simulink model "frbd_64ch_600mhz2"  (R2013b)
(part 3 of 138)

  bus_create0/1(bus_out) -> pipeline599/1(d)
  Constant123/1 -> adcsnap0/3(trig), adcsnap0/2(we)
  pipeline599/1(q) -> adcsnap0/1(din)
  Delay127/1 -> acc_cntrl10/2(sync)
  [acc_len] -> acc_cntrl10/1(acc_len)
  [cnt_rst] -> acc_cntrl10/3(rst)
  Constant124/1 -> acc_len/1(sim_1)
  acc_len/1(in_reg) -> pipeline600/1(d)
  pipeline600/1(q) -> [acc_len]
  Delay119/1 -> pipeline602/1(d)
  pipeline625/1(q) -> simple_bram_vacc86/1(new_acc)
  pipeline617/1(q) -> simple_bram_vacc86/2(din)
  pipeline624/1(q) -> Counter20/1
  acc_cntrl10/1(new_acc) -> pipeline605/1(d), pipeline607/1(d), pipeline603/1(d), pipeline625/1(d), pipeline624/1(d)
  pipeline602/1(q) -> pipeline617/1(d)
  simple_bram_vacc86/1(dout) -> Reinterpret80/1
  spec0/1(data_out) -> Terminator90/1
  Reinterpret80/1 -> spec0/2(data_in)
  simple_bram_vacc86/2(valid) -> Counter20/2, spec0/3(we)
  pipeline603/1(q) -> simple_bram_vacc40/1(new_acc)
  pipeline601/1(q) -> simple_bram_vacc40/2(din)
  simple_bram_vacc40/1(dout) -> Reinterpret81/1
  spec1/1(data_out) -> Terminator83/1
  Reinterpret81/1 -> spec1/2(data_in)
  simple_bram_vacc40/2(valid) -> spec1/3(we)
  pipeline607/1(q) -> simple_bram_vacc42/1(new_acc)
  pipeline606/1(q) -> simple_bram_vacc42/2(din)
  simple_bram_vacc42/1(dout) -> Reinterpret82/1
  spec2/1(data_out) -> Terminator85/1
  Reinterpret82/1 -> spec2/2(data_in)
  simple_bram_vacc42/2(valid) -> spec2/3(we)
  pipeline605/1(q) -> simple_bram_vacc41/1(new_acc)
  pipeline604/1(q) -> simple_bram_vacc41/2(din)
  simple_bram_vacc41/1(dout) -> Reinterpret83/1
  spec3/1(data_out) -> Terminator84/1
  Reinterpret83/1 -> spec3/2(data_in)
  simple_bram_vacc41/2(valid) -> spec3/3(we)
  Counter20/1 -> spec1/1(addr), spec3/1(addr), spec2/1(addr), spec0/1(addr)
  Delay120/1 -> pipeline616/1(d)
  pipeline616/1(q) -> pipeline601/1(d)
  Delay121/1 -> pipeline618/1(d)
  pipeline618/1(q) -> pipeline606/1(d)
  Delay122/1 -> pipeline619/1(d)
  pipeline619/1(q) -> pipeline604/1(d)
  asiaa_adc5g/16(c7) -> Terminator91/1
  asiaa_adc5g/15(c6) -> Terminator92/1
  asiaa_adc5g/14(c5) -> Terminator93/1
  asiaa_adc5g/13(c4) -> Terminator94/1
  asiaa_adc5g/12(c3) -> Terminator95/1
  asiaa_adc5g/11(c2) -> Terminator96/1
  asiaa_adc5g/10(c1) -> Terminator97/1
  asiaa_adc5g/9(c0) -> Terminator98/1
  Constant80/1 -> asiaa_adc5g/2(sim_c)
  Constant1/1 -> asiaa_adc5g/3(sim_sync)
  simple_bram_vacc1/2(valid) -> Terminator18/1
  simple_bram_vacc2/2(valid) -> Terminator1/1
  Constant81/1 -> asiaa_adc5g/1(sim_a)
  Delay5/1 -> acc_cntrl1/2(sync)
  [acc_len2] -> acc_cntrl1/1(acc_len)
  [cnt_rst] -> acc_cntrl1/3(rst)
  Delay8/1 -> pipeline52/1(d)
  pipeline39/1(q) -> simple_bram_vacc7/1(new_acc)
  pipeline30/1(q) -> simple_bram_vacc6/1(new_acc)
  pipeline27/1(q) -> simple_bram_vacc5/1(new_acc)
  pipeline44/1(q) -> simple_bram_vacc4/1(new_acc)
  pipeline12/1(q) -> simple_bram_vacc4/2(din)
  pipeline25/1(q) -> simple_bram_vacc5/2(din)
  pipeline28/1(q) -> simple_bram_vacc6/2(din)
  pipeline38/1(q) -> simple_bram_vacc7/2(din)
  pipeline40/1(q) -> Counter3/1
  simple_bram_vacc4/2(valid) -> pipeline45/1(d), Counter3/2
  simple_bram_vacc4/1(dout) -> Reinterpret4/1
  simple_bram_vacc5/1(dout) -> Reinterpret5/1
  simple_bram_vacc6/1(dout) -> Reinterpret6/1
  simple_bram_vacc7/1(dout) -> Reinterpret7/1
  Reinterpret4/1 -> pipeline43/1(d)
  Reinterpret5/1 -> pipeline46/1(d)
  Reinterpret6/1 -> pipeline47/1(d)
  Reinterpret7/1 -> pipeline48/1(d)
  Counter3/1 -> Relational5/2, Relational4/2
  Constant8/1 -> Mux6/2
  Constant15/1 -> Mux5/2
  Constant16/1 -> Mux7/2
  Constant17/1 -> Mux8/2
  AddSub3/1 -> AddSub5/1
  AddSub4/1 -> AddSub5/2
  pipeline54/1(q) -> pipeline55/1(d)
  edge_detect1/1 -> Logical3/1, Accumulator1/2
  pipeline53/1(q) -> Accumulator1/3, edge_detect1/1
  Slice2/1 -> Accumulator1/1
  Register1/1 -> frb_detector2/1(out_reg)
  [cnt_rst] -> Register1/2
  Relational3/1 -> Register1/1, Register1/3
  simple_bram_vacc7/2(valid) -> Terminator6/1
  pipeline45/1(q) -> Logical4/1, Mux5/1, Mux7/1, Mux8/1, pipeline56/1(d), Parallel_Dedispersor_v1/1(Valid)
  pipeline56/1(q) -> pipeline54/1(d)
  Accumulator1/1 -> Relational3/2, ACC2/2(data_in)
  Counter2/1 -> ACC2/1(addr)
  ACC2/1(data_out) -> Terminator7/1
  Logical3/1 -> Counter2/1
  Delay10/1 -> pipeline49/1(d)
  Delay14/1 -> pipeline50/1(d)
  Delay15/1 -> pipeline51/1(d)
  acc_cntrl1/1(new_acc) -> pipeline40/1(d), pipeline30/1(d), pipeline39/1(d), pipeline27/1(d), pipeline44/1(d)
  pipeline52/1(q) -> pipeline12/1(d)
  pipeline49/1(q) -> pipeline25/1(d)
  pipeline50/1(q) -> pipeline28/1(d)
  pipeline51/1(q) -> pipeline38/1(d)
  pipeline43/1(q) -> Mux6/3
  pipeline46/1(q) -> Mux5/3
  pipeline47/1(q) -> Mux7/3
  pipeline48/1(q) -> Mux8/3
  Mux6/1 -> Parallel_Dedispersor_v1/2(Data1)
  Mux5/1 -> Parallel_Dedispersor_v1/3(Data2)
  Mux7/1 -> Parallel_Dedispersor_v1/4(Data3)
  Mux8/1 -> Parallel_Dedispersor_v1/5(Data4)
  Parallel_Dedispersor_v1/1(Out1) -> pipeline57/1(d)
  Parallel_Dedispersor_v1/2(Out2) -> pipeline58/1(d)
  Parallel_Dedispersor_v1/3(Out3) -> pipeline59/1(d)
  Parallel_Dedispersor_v1/4(Out4) -> pipeline60/1(d)
  pipeline57/1(q) -> AddSub3/1
  pipeline58/1(q) -> AddSub3/2
  pipeline59/1(q) -> AddSub4/1
  pipeline60/1(q) -> AddSub4/2
  pipeline55/1(q) -> pipeline53/1(d)
  AddSub5/1 -> Slice2/1
  pipeline11/1(q) -> Logical4/3
  pipeline10/1(q) -> Logical4/2
  Logical4/1 -> Mux6/1
  Relational4/1 -> pipeline10/1(d)
  Relational5/1 -> pipeline11/1(d)
  Constant2/1 -> Relational4/1
  Constant9/1 -> Relational5/1
  Constant10/1 -> Logical3/2, ACC2/3(we)
  theta2/1(in_reg) -> Convert2/1
  Convert2/1 -> Relational3/1
  simple_bram_vacc5/2(valid) -> Terminator5/1
  simple_bram_vacc6/2(valid) -> Terminator4/1
  Delay19/1 -> acc_cntrl2/2(sync)
  [acc_len3] -> acc_cntrl2/1(acc_len)
  [cnt_rst] -> acc_cntrl2/3(rst)
  Delay21/1 -> pipeline92/1(d)
  pipeline73/1(q) -> simple_bram_vacc11/1(new_acc)
  pipeline71/1(q) -> simple_bram_vacc10/1(new_acc)
  pipeline69/1(q) -> simple_bram_vacc9/1(new_acc)
  pipeline76/1(q) -> simple_bram_vacc8/1(new_acc)
  pipeline66/1(q) -> simple_bram_vacc8/2(din)
  pipeline68/1(q) -> simple_bram_vacc9/2(din)
  pipeline70/1(q) -> simple_bram_vacc10/2(din)
  pipeline72/1(q) -> simple_bram_vacc11/2(din)
  pipeline74/1(q) -> Counter6/1
  simple_bram_vacc8/2(valid) -> pipeline77/1(d), Counter6/2
  simple_bram_vacc8/1(dout) -> Reinterpret8/1
  simple_bram_vacc9/1(dout) -> Reinterpret9/1
  simple_bram_vacc10/1(dout) -> Reinterpret10/1
  simple_bram_vacc11/1(dout) -> Reinterpret11/1
  Reinterpret8/1 -> pipeline75/1(d)
  Reinterpret9/1 -> pipeline78/1(d)
  Reinterpret10/1 -> pipeline80/1(d)
  Reinterpret11/1 -> pipeline83/1(d)
  Counter6/1 -> Relational8/2, Relational7/2
  Constant20/1 -> Mux10/2
  Constant33/1 -> Mux9/2
  Constant34/1 -> Mux11/2
  Constant35/1 -> Mux12/2
  AddSub6/1 -> AddSub8/1
  AddSub7/1 -> AddSub8/2
  pipeline97/1(q) -> pipeline98/1(d)
  edge_detect2/1 -> Logical5/1, Accumulator2/2
  pipeline93/1(q) -> Accumulator2/3, edge_detect2/1
  Slice3/1 -> Accumulator2/1
  Register2/1 -> frb_detector3/1(out_reg)
  [cnt_rst] -> Register2/2
  Relational6/1 -> Register2/1, Register2/3
  simple_bram_vacc11/2(valid) -> Terminator10/1
  pipeline77/1(q) -> Logical6/1, Mux9/1, Mux11/1, Mux12/1, pipeline119/1(d), Parallel_Dedispersor_v4/1(Valid)
  pipeline119/1(q) -> pipeline97/1(d)
  Accumulator2/1 -> Relational6/2, ACC3/2(data_in)
  Counter4/1 -> ACC3/1(addr)
  ACC3/1(data_out) -> Terminator11/1
  Logical5/1 -> Counter4/1
  Delay26/1 -> pipeline85/1(d)
  Delay27/1 -> pipeline90/1(d)
  Delay28/1 -> pipeline91/1(d)
  acc_cntrl2/1(new_acc) -> pipeline74/1(d), pipeline71/1(d), pipeline73/1(d), pipeline69/1(d), pipeline76/1(d)
  pipeline92/1(q) -> pipeline66/1(d)
  pipeline85/1(q) -> pipeline68/1(d)
  pipeline90/1(q) -> pipeline70/1(d)
  pipeline91/1(q) -> pipeline72/1(d)
  pipeline75/1(q) -> Mux10/3
  pipeline78/1(q) -> Mux9/3
  pipeline80/1(q) -> Mux11/3
  pipeline83/1(q) -> Mux12/3
  Mux10/1 -> Parallel_Dedispersor_v4/2(Data1)
  Mux9/1 -> Parallel_Dedispersor_v4/3(Data2)
  Mux11/1 -> Parallel_Dedispersor_v4/4(Data3)
  Mux12/1 -> Parallel_Dedispersor_v4/5(Data4)
  Parallel_Dedispersor_v4/1(Out1) -> pipeline120/1(d)
  Parallel_Dedispersor_v4/2(Out2) -> pipeline121/1(d)
  Parallel_Dedispersor_v4/3(Out3) -> pipeline122/1(d)
  Parallel_Dedispersor_v4/4(Out4) -> pipeline123/1(d)
  pipeline120/1(q) -> AddSub6/1
  pipeline121/1(q) -> AddSub6/2
  pipeline122/1(q) -> AddSub7/1
  pipeline123/1(q) -> AddSub7/2
  pipeline98/1(q) -> pipeline93/1(d)
  AddSub8/1 -> Slice3/1
  pipeline63/1(q) -> Logical6/3
  pipeline62/1(q) -> Logical6/2
  Logical6/1 -> Mux10/1
  Relational7/1 -> pipeline62/1(d)
  Relational8/1 -> pipeline63/1(d)
  Constant19/1 -> Relational7/1
  Constant21/1 -> Relational8/1
  Constant22/1 -> Logical5/2, ACC3/3(we)
  theta3/1(in_reg) -> Convert3/1
  Convert3/1 -> Relational6/1
  simple_bram_vacc9/2(valid) -> Terminator9/1
  simple_bram_vacc10/2(valid) -> Terminator8/1
  Delay29/1 -> acc_cntrl3/2(sync)
  [acc_len4] -> acc_cntrl3/1(acc_len)
  [cnt_rst] -> acc_cntrl3/3(rst)
  Delay30/1 -> pipeline110/1(d)
  pipeline95/1(q) -> simple_bram_vacc15/1(new_acc)
  pipeline84/1(q) -> simple_bram_vacc14/1(new_acc)
  pipeline81/1(q) -> simple_bram_vacc13/1(new_acc)
  pipeline100/1(q) -> simple_bram_vacc12/1(new_acc)
  pipeline65/1(q) -> simple_bram_vacc12/2(din)
  pipeline79/1(q) -> simple_bram_vacc13/2(din)
  pipeline82/1(q) -> simple_bram_vacc14/2(din)
  pipeline94/1(q) -> simple_bram_vacc15/2(din)
  pipeline96/1(q) -> Counter7/1
  simple_bram_vacc12/2(valid) -> Counter7/2, pipeline101/1(d)
  simple_bram_vacc12/1(dout) -> Reinterpret12/1
  simple_bram_vacc13/1(dout) -> Reinterpret13/1
  simple_bram_vacc14/1(dout) -> Reinterpret14/1
  simple_bram_vacc15/1(dout) -> Reinterpret15/1
  Reinterpret12/1 -> pipeline99/1(d)
  Reinterpret13/1 -> pipeline102/1(d)
  Reinterpret14/1 -> pipeline103/1(d)
  Reinterpret15/1 -> pipeline104/1(d)
  Counter7/1 -> Relational10/2, Relational11/2
  Constant36/1 -> Mux14/2
  Constant23/1 -> Mux13/2
  Constant24/1 -> Mux15/2
  Constant25/1 -> Mux16/2
  AddSub9/1 -> AddSub11/1
  AddSub10/1 -> AddSub11/2
  pipeline112/1(q) -> pipeline113/1(d)
  edge_detect3/1 -> Accumulator3/2, Logical7/1
  pipeline111/1(q) -> edge_detect3/1, Accumulator3/3
  Slice4/1 -> Accumulator3/1
  Register3/1 -> frb_detector4/1(out_reg)
  [cnt_rst] -> Register3/2
  Relational9/1 -> Register3/3, Register3/1
  simple_bram_vacc15/2(valid) -> Terminator14/1
  pipeline101/1(q) -> Parallel_Dedispersor_v3/1(Valid), pipeline114/1(d), Mux16/1, Mux15/1, Mux13/1, Logical8/1
  pipeline114/1(q) -> pipeline112/1(d)
  Accumulator3/1 -> ACC4/2(data_in), Relational9/2
  Counter5/1 -> ACC4/1(addr)
  ACC4/1(data_out) -> Terminator15/1
  Logical7/1 -> Counter5/1
  Delay18/1 -> pipeline105/1(d)
  Delay24/1 -> pipeline106/1(d)
  Delay25/1 -> pipeline107/1(d)
  acc_cntrl3/1(new_acc) -> pipeline100/1(d), pipeline81/1(d), pipeline95/1(d), pipeline84/1(d), pipeline96/1(d)
  pipeline110/1(q) -> pipeline65/1(d)
  pipeline105/1(q) -> pipeline79/1(d)
  pipeline106/1(q) -> pipeline82/1(d)
  pipeline107/1(q) -> pipeline94/1(d)
  pipeline99/1(q) -> Mux14/3
  pipeline102/1(q) -> Mux13/3
  pipeline103/1(q) -> Mux15/3
  pipeline104/1(q) -> Mux16/3
  Mux14/1 -> Parallel_Dedispersor_v3/2(Data1)
  Mux13/1 -> Parallel_Dedispersor_v3/3(Data2)
  Mux15/1 -> Parallel_Dedispersor_v3/4(Data3)
  Mux16/1 -> Parallel_Dedispersor_v3/5(Data4)
  Parallel_Dedispersor_v3/1(Out1) -> pipeline115/1(d)
  Parallel_Dedispersor_v3/2(Out2) -> pipeline116/1(d)
  Parallel_Dedispersor_v3/3(Out3) -> pipeline117/1(d)
  Parallel_Dedispersor_v3/4(Out4) -> pipeline118/1(d)
  pipeline115/1(q) -> AddSub9/1
  pipeline116/1(q) -> AddSub9/2
  pipeline117/1(q) -> AddSub10/1
  pipeline118/1(q) -> AddSub10/2
  pipeline113/1(q) -> pipeline111/1(d)
  AddSub11/1 -> Slice4/1
  pipeline64/1(q) -> Logical8/3
  pipeline61/1(q) -> Logical8/2
  Logical8/1 -> Mux14/1
  Relational10/1 -> pipeline61/1(d)
  Relational11/1 -> pipeline64/1(d)
  Constant32/1 -> Relational10/1
  Constant37/1 -> Relational11/1
  Constant18/1 -> ACC4/3(we), Logical7/2
  theta4/1(in_reg) -> Convert4/1
  Convert4/1 -> Relational9/1
  simple_bram_vacc13/2(valid) -> Terminator13/1
  simple_bram_vacc14/2(valid) -> Terminator12/1
  Delay32/1 -> acc_cntrl4/2(sync)
  [acc_len5] -> acc_cntrl4/1(acc_len)
  [cnt_rst] -> acc_cntrl4/3(rst)
  Delay39/1 -> pipeline178/1(d)
  pipeline163/1(q) -> simple_bram_vacc25/1(new_acc)
  pipeline161/1(q) -> simple_bram_vacc24/1(new_acc)
  pipeline159/1(q) -> simple_bram_vacc17/1(new_acc)
  pipeline166/1(q) -> simple_bram_vacc16/1(new_acc)
  pipeline157/1(q) -> simple_bram_vacc16/2(din)
  pipeline158/1(q) -> simple_bram_vacc17/2(din)
  pipeline160/1(q) -> simple_bram_vacc24/2(din)
  pipeline162/1(q) -> simple_bram_vacc25/2(din)
  pipeline164/1(q) -> Counter10/1
  simple_bram_vacc16/2(valid) -> pipeline167/1(d), Counter10/2
  simple_bram_vacc16/1(dout) -> Reinterpret16/1
  simple_bram_vacc17/1(dout) -> Reinterpret17/1
  simple_bram_vacc24/1(dout) -> Reinterpret24/1
  simple_bram_vacc25/1(dout) -> Reinterpret25/1
  Reinterpret16/1 -> pipeline165/1(d)
  Reinterpret17/1 -> pipeline168/1(d)
  Reinterpret24/1 -> pipeline170/1(d)
  Reinterpret25/1 -> pipeline173/1(d)
  Counter10/1 -> Relational16/2, Relational13/2
  Constant40/1 -> Mux25/2
  Constant61/1 -> Mux17/2
  Constant62/1 -> Mux26/2
  Constant63/1 -> Mux27/2
  AddSub12/1 -> AddSub16/1
  AddSub13/1 -> AddSub16/2
  pipeline183/1(q) -> pipeline184/1(d)
  edge_detect4/1 -> Logical9/1, Accumulator4/2
  pipeline179/1(q) -> Accumulator4/3, edge_detect4/1
  Slice5/1 -> Accumulator4/1
  Register4/1 -> frb_detector5/1(out_reg)
  [cnt_rst] -> Register4/2
  Relational12/1 -> Register4/1, Register4/3
  simple_bram_vacc25/2(valid) -> Terminator27/1
  pipeline167/1(q) -> Logical10/1, Mux17/1, Mux26/1, Mux27/1, pipeline209/1(d), Parallel_Dedispersor_v6/1(Valid)
  pipeline209/1(q) -> pipeline183/1(d)
  Accumulator4/1 -> Relational12/2, ACC5/2(data_in)
  Counter8/1 -> ACC5/1(addr)
  ACC5/1(data_out) -> Terminator28/1
  Logical9/1 -> Counter8/1
  Delay52/1 -> pipeline175/1(d)
  Delay53/1 -> pipeline176/1(d)
  Delay54/1 -> pipeline177/1(d)
  acc_cntrl4/1(new_acc) -> pipeline164/1(d), pipeline161/1(d), pipeline163/1(d), pipeline159/1(d), pipeline166/1(d)
  pipeline178/1(q) -> pipeline157/1(d)
  pipeline175/1(q) -> pipeline158/1(d)
  pipeline176/1(q) -> pipeline160/1(d)
  pipeline177/1(q) -> pipeline162/1(d)
  pipeline165/1(q) -> Mux25/3
  pipeline168/1(q) -> Mux17/3
  pipeline170/1(q) -> Mux26/3
  pipeline173/1(q) -> Mux27/3
  Mux25/1 -> Parallel_Dedispersor_v6/2(Data1)
  Mux17/1 -> Parallel_Dedispersor_v6/3(Data2)
  Mux26/1 -> Parallel_Dedispersor_v6/4(Data3)
  Mux27/1 -> Parallel_Dedispersor_v6/5(Data4)
  Parallel_Dedispersor_v6/1(Out1) -> pipeline228/1(d)
  Parallel_Dedispersor_v6/2(Out2) -> pipeline229/1(d)
  Parallel_Dedispersor_v6/3(Out3) -> pipeline230/1(d)
  Parallel_Dedispersor_v6/4(Out4) -> pipeline231/1(d)
  pipeline228/1(q) -> AddSub12/1
  pipeline229/1(q) -> AddSub12/2
  pipeline230/1(q) -> AddSub13/1
  pipeline231/1(q) -> AddSub13/2
  pipeline184/1(q) -> pipeline179/1(d)
  AddSub16/1 -> Slice5/1
  pipeline140/1(q) -> Logical10/3
  pipeline133/1(q) -> Logical10/2
  Logical10/1 -> Mux25/1
  Relational13/1 -> pipeline133/1(d)
  Relational16/1 -> pipeline140/1(d)
  Constant39/1 -> Relational13/1
  Constant41/1 -> Relational16/1
  Constant42/1 -> Logical9/2, ACC5/3(we)
  theta5/1(in_reg) -> Convert5/1
  Convert5/1 -> Relational12/1
  Delay3/1 -> Delay5/1, Delay19/1, Delay29/1, Delay32/1, Delay55/1, Delay43/1, Delay50/1, Delay58/1, Delay65/1, Delay127/1, Delay12/1
  simple_bram_vacc17/2(valid) -> Terminator26/1
  simple_bram_vacc24/2(valid) -> Terminator16/1
  power7/1 -> Delay15/1, Delay28/1, Delay25/1, Delay54/1, Delay41/1, Delay49/1, Delay46/1, Delay64/1, Delay61/1, Delay122/1, Delay37/1
  power5/1 -> Delay10/1, Delay26/1, Delay52/1, Delay31/1, Delay42/1, Delay62/1, Delay57/1, Delay120/1, Delay47/1, Delay18/1, Delay33/1
  Delay55/1 -> acc_cntrl5/2(sync)
  [acc_len6] -> acc_cntrl5/1(acc_len)
  [cnt_rst] -> acc_cntrl5/3(rst)
  Delay56/1 -> pipeline194/1(d)
  pipeline181/1(q) -> simple_bram_vacc29/1(new_acc)
  pipeline174/1(q) -> simple_bram_vacc28/1(new_acc)
  pipeline171/1(q) -> simple_bram_vacc27/1(new_acc)
  pipeline186/1(q) -> simple_bram_vacc26/1(new_acc)
  pipeline152/1(q) -> simple_bram_vacc26/2(din)
  pipeline169/1(q) -> simple_bram_vacc27/2(din)
  pipeline172/1(q) -> simple_bram_vacc28/2(din)
  pipeline180/1(q) -> simple_bram_vacc29/2(din)
  pipeline182/1(q) -> Counter11/1
  simple_bram_vacc26/2(valid) -> Counter11/2, pipeline187/1(d)
  simple_bram_vacc26/1(dout) -> Reinterpret26/1
  simple_bram_vacc27/1(dout) -> Reinterpret27/1
  simple_bram_vacc28/1(dout) -> Reinterpret28/1
  simple_bram_vacc29/1(dout) -> Reinterpret29/1
  Reinterpret26/1 -> pipeline185/1(d)
  Reinterpret27/1 -> pipeline188/1(d)
  Reinterpret28/1 -> pipeline189/1(d)
  Reinterpret29/1 -> pipeline190/1(d)
  Counter11/1 -> Relational18/2, Relational19/2
  Constant64/1 -> Mux29/2
  Constant43/1 -> Mux28/2
  Constant44/1 -> Mux30/2
  Constant45/1 -> Mux31/2
  AddSub17/1 -> AddSub19/1
  AddSub18/1 -> AddSub19/2
  pipeline196/1(q) -> pipeline197/1(d)
  edge_detect5/1 -> Accumulator5/2, Logical11/1
  pipeline195/1(q) -> edge_detect5/1, Accumulator5/3
  Slice6/1 -> Accumulator5/1
  Register5/1 -> frb_detector6/1(out_reg)
  [cnt_rst] -> Register5/2
  Relational17/1 -> Register5/3, Register5/1
  simple_bram_vacc29/2(valid) -> Terminator31/1
  pipeline187/1(q) -> Parallel_Dedispersor_v5/1(Valid), pipeline198/1(d), Mux31/1, Mux30/1, Mux28/1, Logical12/1
  pipeline198/1(q) -> pipeline196/1(d)
  Accumulator5/1 -> ACC6/2(data_in), Relational17/2
  Counter9/1 -> ACC6/1(addr)
  ACC6/1(data_out) -> Terminator32/1
  Logical11/1 -> Counter9/1
  Delay31/1 -> pipeline191/1(d)
  Delay40/1 -> pipeline192/1(d)
  Delay41/1 -> pipeline193/1(d)
  acc_cntrl5/1(new_acc) -> pipeline186/1(d), pipeline171/1(d), pipeline181/1(d), pipeline174/1(d), pipeline182/1(d)
  pipeline194/1(q) -> pipeline152/1(d)
  pipeline191/1(q) -> pipeline169/1(d)
  pipeline192/1(q) -> pipeline172/1(d)
  pipeline193/1(q) -> pipeline180/1(d)
  pipeline185/1(q) -> Mux29/3
  pipeline188/1(q) -> Mux28/3
  pipeline189/1(q) -> Mux30/3
  pipeline190/1(q) -> Mux31/3
  Mux29/1 -> Parallel_Dedispersor_v5/2(Data1)
  Mux28/1 -> Parallel_Dedispersor_v5/3(Data2)
  Mux30/1 -> Parallel_Dedispersor_v5/4(Data3)
  Mux31/1 -> Parallel_Dedispersor_v5/5(Data4)
  Parallel_Dedispersor_v5/1(Out1) -> pipeline199/1(d)
  Parallel_Dedispersor_v5/2(Out2) -> pipeline200/1(d)
  Parallel_Dedispersor_v5/3(Out3) -> pipeline201/1(d)
  Parallel_Dedispersor_v5/4(Out4) -> pipeline202/1(d)
  pipeline199/1(q) -> AddSub17/1
  pipeline200/1(q) -> AddSub17/2
  pipeline201/1(q) -> AddSub18/1
  pipeline202/1(q) -> AddSub18/2
  pipeline197/1(q) -> pipeline195/1(d)
  AddSub19/1 -> Slice6/1
  pipeline141/1(q) -> Logical12/3
  pipeline124/1(q) -> Logical12/2
  Logical12/1 -> Mux29/1
  Relational18/1 -> pipeline124/1(d)
  Relational19/1 -> pipeline141/1(d)
  Constant48/1 -> Relational18/1
  Constant65/1 -> Relational19/1
  Constant38/1 -> ACC6/3(we), Logical11/2
  theta6/1(in_reg) -> Convert6/1
  Convert6/1 -> Relational17/1
  simple_bram_vacc27/2(valid) -> Terminator30/1
  simple_bram_vacc28/2(valid) -> Terminator29/1
  Delay43/1 -> acc_cntrl6/2(sync)
  [acc_len7] -> acc_cntrl6/1(acc_len)
  [cnt_rst] -> acc_cntrl6/3(rst)
  Delay44/1 -> pipeline234/1(d)
  pipeline215/1(q) -> simple_bram_vacc19/1(new_acc)
  pipeline213/1(q) -> simple_bram_vacc18/1(new_acc)
  pipeline211/1(q) -> simple_bram_vacc31/1(new_acc)
  pipeline218/1(q) -> simple_bram_vacc30/1(new_acc)
  pipeline208/1(q) -> simple_bram_vacc30/2(din)
  pipeline210/1(q) -> simple_bram_vacc31/2(din)
  pipeline212/1(q) -> simple_bram_vacc18/2(din)
  pipeline214/1(q) -> simple_bram_vacc19/2(din)
  pipeline216/1(q) -> Counter14/1
  simple_bram_vacc30/2(valid) -> Counter14/2, pipeline219/1(d)
  simple_bram_vacc30/1(dout) -> Reinterpret30/1
  simple_bram_vacc31/1(dout) -> Reinterpret31/1
  simple_bram_vacc18/1(dout) -> Reinterpret18/1
  simple_bram_vacc19/1(dout) -> Reinterpret19/1
  Reinterpret30/1 -> pipeline217/1(d)
  Reinterpret31/1 -> pipeline220/1(d)
  Reinterpret18/1 -> pipeline222/1(d)
  Reinterpret19/1 -> pipeline225/1(d)
  Counter14/1 -> Relational21/2, Relational22/2
  Constant49/1 -> Mux18/2
  Constant56/1 -> Mux32/2
  Constant57/1 -> Mux19/2
  Constant58/1 -> Mux20/2
  AddSub20/1 -> AddSub22/1
  AddSub21/1 -> AddSub22/2
  pipeline239/1(q) -> pipeline240/1(d)
  edge_detect6/1 -> Accumulator6/2, Logical13/1
  pipeline235/1(q) -> edge_detect6/1, Accumulator6/3
  Slice7/1 -> Accumulator6/1
  Register6/1 -> frb_detector7/1(out_reg)
  [cnt_rst] -> Register6/2
  Relational20/1 -> Register6/3, Register6/1
  simple_bram_vacc19/2(valid) -> Terminator17/1
  pipeline219/1(q) -> Parallel_Dedispersor_v8/1(Valid), pipeline151/1(d), Mux20/1, Mux19/1, Mux32/1, Logical14/1
  pipeline151/1(q) -> pipeline239/1(d)
  Accumulator6/1 -> ACC7/2(data_in), Relational20/2
  Counter12/1 -> ACC7/1(addr)
  ACC7/1(data_out) -> Terminator19/1
  Logical13/1 -> Counter12/1
  Delay47/1 -> pipeline227/1(d)
  Delay48/1 -> pipeline232/1(d)
  Delay49/1 -> pipeline233/1(d)
  acc_cntrl6/1(new_acc) -> pipeline218/1(d), pipeline211/1(d), pipeline215/1(d), pipeline213/1(d), pipeline216/1(d)
  pipeline234/1(q) -> pipeline208/1(d)
  pipeline227/1(q) -> pipeline210/1(d)
  pipeline232/1(q) -> pipeline212/1(d)
  pipeline233/1(q) -> pipeline214/1(d)
  pipeline217/1(q) -> Mux18/3
  pipeline220/1(q) -> Mux32/3
  pipeline222/1(q) -> Mux19/3
  pipeline225/1(q) -> Mux20/3
  Mux18/1 -> Parallel_Dedispersor_v8/2(Data1)
  Mux32/1 -> Parallel_Dedispersor_v8/3(Data2)
  Mux19/1 -> Parallel_Dedispersor_v8/4(Data3)
  Mux20/1 -> Parallel_Dedispersor_v8/5(Data4)
  Parallel_Dedispersor_v8/1(Out1) -> pipeline153/1(d)
  Parallel_Dedispersor_v8/2(Out2) -> pipeline154/1(d)
  Parallel_Dedispersor_v8/3(Out3) -> pipeline155/1(d)
  Parallel_Dedispersor_v8/4(Out4) -> pipeline156/1(d)
  pipeline153/1(q) -> AddSub20/1
  pipeline154/1(q) -> AddSub20/2
  pipeline155/1(q) -> AddSub21/1
  pipeline156/1(q) -> AddSub21/2
  pipeline240/1(q) -> pipeline235/1(d)
  AddSub22/1 -> Slice7/1
  pipeline205/1(q) -> Logical14/3
  pipeline204/1(q) -> Logical14/2
  Logical14/1 -> Mux18/1
  Relational21/1 -> pipeline204/1(d)
  Relational22/1 -> pipeline205/1(d)
  Constant47/1 -> Relational21/1
  Constant50/1 -> Relational22/1
  Constant51/1 -> ACC7/3(we), Logical13/2
  theta7/1(in_reg) -> Convert7/1
  Convert7/1 -> Relational20/1
  simple_bram_vacc31/2(valid) -> Terminator34/1
  simple_bram_vacc18/2(valid) -> Terminator33/1
  Delay50/1 -> acc_cntrl7/2(sync)
  [acc_len8] -> acc_cntrl7/1(acc_len)
  [cnt_rst] -> acc_cntrl7/3(rst)
  Delay51/1 -> pipeline142/1(d)
  pipeline237/1(q) -> simple_bram_vacc23/1(new_acc)
  pipeline226/1(q) -> simple_bram_vacc22/1(new_acc)
  pipeline223/1(q) -> simple_bram_vacc21/1(new_acc)
  pipeline125/1(q) -> simple_bram_vacc20/1(new_acc)
  pipeline207/1(q) -> simple_bram_vacc20/2(din)
  pipeline221/1(q) -> simple_bram_vacc21/2(din)
  pipeline224/1(q) -> simple_bram_vacc22/2(din)
  pipeline236/1(q) -> simple_bram_vacc23/2(din)
  pipeline238/1(q) -> Counter15/1
  simple_bram_vacc20/2(valid) -> pipeline126/1(d), Counter15/2
  simple_bram_vacc20/1(dout) -> Reinterpret20/1
  simple_bram_vacc21/1(dout) -> Reinterpret21/1
  simple_bram_vacc22/1(dout) -> Reinterpret22/1
  simple_bram_vacc23/1(dout) -> Reinterpret23/1
  Reinterpret20/1 -> pipeline241/1(d)
  Reinterpret21/1 -> pipeline127/1(d)
  Reinterpret22/1 -> pipeline128/1(d)
  Reinterpret23/1 -> pipeline129/1(d)
  Counter15/1 -> Relational15/2, Relational14/2
  Constant59/1 -> Mux22/2
  Constant52/1 -> Mux21/2
  Constant53/1 -> Mux23/2
  Constant54/1 -> Mux24/2
  AddSub23/1 -> AddSub15/1
  AddSub14/1 -> AddSub15/2
  pipeline144/1(q) -> pipeline145/1(d)
  edge_detect7/1 -> Logical15/1, Accumulator7/2
  pipeline143/1(q) -> Accumulator7/3, edge_detect7/1
  Slice8/1 -> Accumulator7/1
  Register7/1 -> frb_detector8/1(out_reg)
  [cnt_rst] -> Register7/2
  Relational23/1 -> Register7/1, Register7/3
  simple_bram_vacc23/2(valid) -> Terminator24/1
  pipeline126/1(q) -> Logical16/1, Mux21/1, Mux23/1, Mux24/1, pipeline146/1(d), Parallel_Dedispersor_v7/1(Valid)
  pipeline146/1(q) -> pipeline144/1(d)
  Accumulator7/1 -> Relational23/2, ACC8/2(data_in)
  Counter13/1 -> ACC8/1(addr)
  ACC8/1(data_out) -> Terminator25/1
  Logical15/1 -> Counter13/1
  Delay42/1 -> pipeline130/1(d)
  Delay45/1 -> pipeline131/1(d)
  Delay46/1 -> pipeline132/1(d)
  acc_cntrl7/1(new_acc) -> pipeline238/1(d), pipeline226/1(d), pipeline237/1(d), pipeline223/1(d), pipeline125/1(d)
  pipeline142/1(q) -> pipeline207/1(d)
  pipeline130/1(q) -> pipeline221/1(d)
  pipeline131/1(q) -> pipeline224/1(d)
  pipeline132/1(q) -> pipeline236/1(d)
  pipeline241/1(q) -> Mux22/3
  pipeline127/1(q) -> Mux21/3
  pipeline128/1(q) -> Mux23/3
  pipeline129/1(q) -> Mux24/3
  Mux22/1 -> Parallel_Dedispersor_v7/2(Data1)
  Mux21/1 -> Parallel_Dedispersor_v7/3(Data2)
  Mux23/1 -> Parallel_Dedispersor_v7/4(Data3)
  Mux24/1 -> Parallel_Dedispersor_v7/5(Data4)
  Parallel_Dedispersor_v7/1(Out1) -> pipeline147/1(d)
  Parallel_Dedispersor_v7/2(Out2) -> pipeline148/1(d)
  Parallel_Dedispersor_v7/3(Out3) -> pipeline149/1(d)
  Parallel_Dedispersor_v7/4(Out4) -> pipeline150/1(d)
  pipeline147/1(q) -> AddSub23/1
  pipeline148/1(q) -> AddSub23/2
  pipeline149/1(q) -> AddSub14/1
  pipeline150/1(q) -> AddSub14/2
  pipeline145/1(q) -> pipeline143/1(d)
  AddSub15/1 -> Slice8/1
  pipeline206/1(q) -> Logical16/3
  pipeline203/1(q) -> Logical16/2
  Logical16/1 -> Mux22/1
  Relational14/1 -> pipeline203/1(d)
  Relational15/1 -> pipeline206/1(d)
  Constant55/1 -> Relational14/1
  Constant60/1 -> Relational15/1
  Constant46/1 -> Logical15/2, ACC8/3(we)
  theta8/1(in_reg) -> Convert8/1
  Convert8/1 -> Relational23/1
  simple_bram_vacc21/2(valid) -> Terminator23/1
  simple_bram_vacc22/2(valid) -> Terminator20/1
  Delay58/1 -> acc_cntrl8/2(sync)
  [acc_len9] -> acc_cntrl8/1(acc_len)
  [cnt_rst] -> acc_cntrl8/3(rst)
  Delay59/1 -> pipeline290/1(d)
  pipeline275/1(q) -> simple_bram_vacc33/1(new_acc)
  pipeline273/1(q) -> simple_bram_vacc32/1(new_acc)
  pipeline271/1(q) -> simple_bram_vacc39/1(new_acc)
  pipeline278/1(q) -> simple_bram_vacc38/1(new_acc)
  pipeline269/1(q) -> simple_bram_vacc38/2(din)
  pipeline270/1(q) -> simple_bram_vacc39/2(din)
  pipeline272/1(q) -> simple_bram_vacc32/2(din)
  pipeline274/1(q) -> simple_bram_vacc33/2(din)
  pipeline276/1(q) -> Counter18/1
  simple_bram_vacc38/2(valid) -> pipeline279/1(d), Counter18/2
  simple_bram_vacc38/1(dout) -> Reinterpret38/1
  simple_bram_vacc39/1(dout) -> Reinterpret39/1
  simple_bram_vacc32/1(dout) -> Reinterpret32/1
  simple_bram_vacc33/1(dout) -> Reinterpret33/1
  Reinterpret38/1 -> pipeline277/1(d)
  Reinterpret39/1 -> pipeline280/1(d)
  Reinterpret32/1 -> pipeline282/1(d)
  Reinterpret33/1 -> pipeline285/1(d)
  Counter18/1 -> Relational28/2, Relational27/2
  Constant68/1 -> Mux33/2
  Constant75/1 -> Mux40/2
  Constant76/1 -> Mux34/2
  Constant77/1 -> Mux35/2
  AddSub26/1 -> AddSub28/1
  AddSub27/1 -> AddSub28/2
  pipeline295/1(q) -> pipeline296/1(d)
  edge_detect8/1 -> Logical17/1, Accumulator8/2
  pipeline291/1(q) -> Accumulator8/3, edge_detect8/1
  Slice9/1 -> Accumulator8/1
  Register8/1 -> frb_detector9/1(out_reg)
  [cnt_rst] -> Register8/2
  Relational26/1 -> Register8/1, Register8/3
  simple_bram_vacc33/2(valid) -> Terminator35/1
  pipeline279/1(q) -> Mux40/1, Mux34/1, Mux35/1, pipeline259/1(d), Parallel_Dedispersor_v10/1(Valid), Logical18/1
  pipeline259/1(q) -> pipeline295/1(d)
  Accumulator8/1 -> Relational26/2, ACC9/2(data_in)
  Counter16/1 -> ACC9/1(addr)
  ACC9/1(data_out) -> Terminator36/1
  Logical17/1 -> Counter16/1
  Delay62/1 -> pipeline287/1(d)
  Delay63/1 -> pipeline288/1(d)
  Delay64/1 -> pipeline289/1(d)
  acc_cntrl8/1(new_acc) -> pipeline276/1(d), pipeline273/1(d), pipeline275/1(d), pipeline271/1(d), pipeline278/1(d)
  pipeline290/1(q) -> pipeline269/1(d)
  pipeline287/1(q) -> pipeline270/1(d)
  pipeline288/1(q) -> pipeline272/1(d)
  pipeline289/1(q) -> pipeline274/1(d)
  pipeline277/1(q) -> Mux33/3
  pipeline280/1(q) -> Mux40/3
  pipeline282/1(q) -> Mux34/3
  pipeline285/1(q) -> Mux35/3
  Mux33/1 -> Parallel_Dedispersor_v10/2(Data1)
  Mux40/1 -> Parallel_Dedispersor_v10/3(Data2)
  Mux34/1 -> Parallel_Dedispersor_v10/4(Data3)
  Mux35/1 -> Parallel_Dedispersor_v10/5(Data4)
  Parallel_Dedispersor_v10/1(Out1) -> pipeline260/1(d)
  Parallel_Dedispersor_v10/2(Out2) -> pipeline261/1(d)
  Parallel_Dedispersor_v10/3(Out3) -> pipeline262/1(d)
  Parallel_Dedispersor_v10/4(Out4) -> pipeline263/1(d)
  pipeline260/1(q) -> AddSub26/1
  pipeline261/1(q) -> AddSub26/2
  pipeline262/1(q) -> AddSub27/1
  pipeline263/1(q) -> AddSub27/2
  pipeline296/1(q) -> pipeline291/1(d)
  AddSub28/1 -> Slice9/1
  pipeline266/1(q) -> Logical18/3
  pipeline265/1(q) -> Logical18/2
  Logical18/1 -> Mux33/1
  Relational27/1 -> pipeline265/1(d)
  Relational28/1 -> pipeline266/1(d)
  Constant67/1 -> Relational27/1
  Constant69/1 -> Relational28/1
  Constant70/1 -> Logical17/2, ACC9/3(we)
  theta9/1(in_reg) -> Convert9/1
  Convert9/1 -> Relational26/1
  simple_bram_vacc39/2(valid) -> Terminator42/1
  simple_bram_vacc32/2(valid) -> Terminator41/1
  Delay65/1 -> acc_cntrl9/2(sync)
  [acc_len10] -> acc_cntrl9/1(acc_len)
  [cnt_rst] -> acc_cntrl9/3(rst)
  Delay66/1 -> pipeline250/1(d)
  pipeline293/1(q) -> simple_bram_vacc37/1(new_acc)
  pipeline286/1(q) -> simple_bram_vacc36/1(new_acc)
  pipeline283/1(q) -> simple_bram_vacc35/1(new_acc)
  pipeline242/1(q) -> simple_bram_vacc34/1(new_acc)
  pipeline268/1(q) -> simple_bram_vacc34/2(din)
  pipeline281/1(q) -> simple_bram_vacc35/2(din)
  pipeline284/1(q) -> simple_bram_vacc36/2(din)
  pipeline292/1(q) -> simple_bram_vacc37/2(din)
  pipeline294/1(q) -> Counter19/1
  simple_bram_vacc34/2(valid) -> Counter19/2, pipeline243/1(d)
  simple_bram_vacc34/1(dout) -> Reinterpret34/1
  simple_bram_vacc35/1(dout) -> Reinterpret35/1
  simple_bram_vacc36/1(dout) -> Reinterpret36/1
  simple_bram_vacc37/1(dout) -> Reinterpret37/1
  Reinterpret34/1 -> pipeline297/1(d)
  Reinterpret35/1 -> pipeline244/1(d)
  Reinterpret36/1 -> pipeline245/1(d)
  Reinterpret37/1 -> pipeline246/1(d)
  Counter19/1 -> Relational24/2, Relational25/2
  Constant78/1 -> Mux37/2
  Constant71/1 -> Mux36/2
  Constant72/1 -> Mux38/2
  Constant73/1 -> Mux39/2
  AddSub29/1 -> AddSub25/1
  AddSub24/1 -> AddSub25/2
  pipeline252/1(q) -> pipeline253/1(d)
  edge_detect9/1 -> Accumulator9/2, Logical19/1
  pipeline251/1(q) -> edge_detect9/1, Accumulator9/3
  Slice10/1 -> Accumulator9/1
  Register9/1 -> frb_detector10/1(out_reg)
  [cnt_rst] -> Register9/2
  Relational29/1 -> Register9/3, Register9/1
  simple_bram_vacc37/2(valid) -> Terminator39/1
  pipeline243/1(q) -> Parallel_Dedispersor_v9/1(Valid), pipeline254/1(d), Mux39/1, Mux38/1, Mux36/1, Logical20/1
  pipeline254/1(q) -> pipeline252/1(d)
  Accumulator9/1 -> ACC10/2(data_in), Relational29/2
  Counter17/1 -> ACC10/1(addr)
  ACC10/1(data_out) -> Terminator40/1
  Logical19/1 -> Counter17/1
  Delay57/1 -> pipeline247/1(d)
  Delay60/1 -> pipeline248/1(d)
  Delay61/1 -> pipeline249/1(d)
  acc_cntrl9/1(new_acc) -> pipeline242/1(d), pipeline283/1(d), pipeline293/1(d), pipeline286/1(d), pipeline294/1(d)
  pipeline250/1(q) -> pipeline268/1(d)
  pipeline247/1(q) -> pipeline281/1(d)
  pipeline248/1(q) -> pipeline284/1(d)
  pipeline249/1(q) -> pipeline292/1(d)
  pipeline297/1(q) -> Mux37/3
  pipeline244/1(q) -> Mux36/3
  pipeline245/1(q) -> Mux38/3
  pipeline246/1(q) -> Mux39/3
  Mux37/1 -> Parallel_Dedispersor_v9/2(Data1)
  Mux36/1 -> Parallel_Dedispersor_v9/3(Data2)
  Mux38/1 -> Parallel_Dedispersor_v9/4(Data3)
  Mux39/1 -> Parallel_Dedispersor_v9/5(Data4)
  Parallel_Dedispersor_v9/1(Out1) -> pipeline255/1(d)
  Parallel_Dedispersor_v9/2(Out2) -> pipeline256/1(d)
  Parallel_Dedispersor_v9/3(Out3) -> pipeline257/1(d)
  Parallel_Dedispersor_v9/4(Out4) -> pipeline258/1(d)
  pipeline255/1(q) -> AddSub29/1
  pipeline256/1(q) -> AddSub29/2
  pipeline257/1(q) -> AddSub24/1
  pipeline258/1(q) -> AddSub24/2
  pipeline253/1(q) -> pipeline251/1(d)
  AddSub25/1 -> Slice10/1
  pipeline267/1(q) -> Logical20/3
  pipeline264/1(q) -> Logical20/2
  Logical20/1 -> Mux37/1
  Relational24/1 -> pipeline264/1(d)
  Relational25/1 -> pipeline267/1(d)
  Constant74/1 -> Relational24/1
  Constant79/1 -> Relational25/1
  Constant66/1 -> ACC10/3(we), Logical19/2
  theta10/1(in_reg) -> Convert10/1
  Convert10/1 -> Relational29/1
  simple_bram_vacc35/2(valid) -> Terminator38/1
  simple_bram_vacc36/2(valid) -> Terminator37/1
  power1/1 -> Delay8/1, Delay21/1, Delay30/1, Delay39/1, Delay56/1, Delay44/1, Delay51/1, Delay59/1, Delay66/1, Delay119/1, Delay13/1
  power6/1 -> Delay14/1, Delay27/1, Delay24/1, Delay53/1, Delay40/1, Delay45/1, Delay63/1, Delay60/1, Delay121/1, Delay48/1, Delay35/1
